simulink model "NonLin_BicycleModelSimulink"  (R2017b)
settings: Solver=VariableStepAuto  StartTime=0.0  StopTime=5  FixedStep=0.001  MaxStep=0.010  MinStep=0.005  RelTol=1e-3  EnableMultiTasking=on
values from neighbouring files (symbols this model uses):
  a = L*weight_dist    (= 0.762)    [BicycleModel.m]    (also in BicycleModelSim.m = 1.1; BicycleModelSimv2.m = 0.4572; FullCarModel.m = 0.6096; NonLin_BicycleModel.m = 0.8382)
  b = L*(1-weight_dist)    (= 0.762)    [BicycleModel.m]    (also in BicycleModelSim.m = 1.6; BicycleModelSimv2.m = 1.0668; FullCarModel.m = 0.9144; NonLin_BicycleModel.m = 0.6858)
  I_zz = 83.28    [BicycleModel.m]    (also in BicycleModelSim.m = 2500; BicycleModelSimv2.m; FullCarModel.m; NonLin_BicycleModel.m)
  m = 535*0.453592    (= 242.67172)    [BicycleModel.m]    (also in BicycleModelSim.m = 1500; BicycleModelSimv2.m = 242.6718; FullCarModel.m = 242.6718; NonLin_BicycleModel.m = 242.6718)
  step_steer = 1    [BicycleModelSimv2.m]    (also in FullCarModel.m = 0.0523598775598; NonLin_BicycleModel.m = 0.12217304764)
  weight_dist = 0.5    [BicycleModel.m]    (also in BicycleModelSimv2.m = 0.3; FullCarModel.m = 0.4; NonLin_BicycleModel.m = 0.55; ResponseTimePlotter.m = 0.51)
  X = cell2mat(Xbestcell)    [FullCarModel.m]    (also in NonLin_BicycleModel.m)
settings Model: Creator=tonylu  LastModifiedBy=tonylu
settings OptimizationCC: LifeSpan=inf
settings DebuggingCC: SFUnexpectedBacktrackingDiag=warning  SFNoUnconditionalDefaultTransitionDiag=warning  SFExecutionAtInitializationDiag=none
settings CodeAppCC: StateflowObjectComments=on
settings GRTTargetCC: TargetLangStandard=C89/C90 (ANSI)  GeneratePreprocessorConditionals=Disable all
settings ConfigComp: CovMetricSettings=dw  CovHtmlReporting=on  CovSaveCumulativeToWorkspaceVar=on  CovSaveSingleToWorkspaceVar=on  CovExternalEMLEnable=off

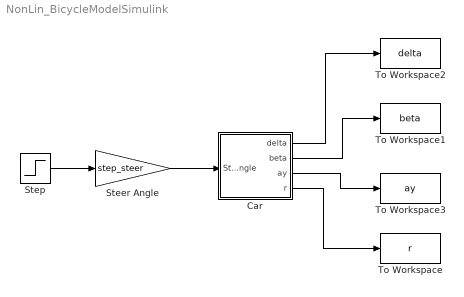
== system NonLin_BicycleModelSimulink ==
  Car : Subsystem
  Steer Angle : Gain  Gain=step_steer
  Step : Step  Time=0  SampleTime=0
  To Workspace : ToWorkspace  VariableName=r  SaveFormat=Structure With Time  SampleTime=0.01
  To Workspace1 : ToWorkspace  VariableName=beta  SaveFormat=Structure With Time  SampleTime=0.01
  To Workspace2 : ToWorkspace  VariableName=delta  SaveFormat=Structure With Time  SampleTime=0.01
  To Workspace3 : ToWorkspace  VariableName=ay  SaveFormat=Structure With Time  SampleTime=0.01
  wires:
  Car/1(delta) -> To Workspace2/1
  Car/2(beta) -> To Workspace1/1
  Car/3(ay) -> To Workspace3/1
  Car/4(r) -> To Workspace/1
  Steer Angle/1 -> Car/1(Steer Angle)
  Step/1 -> Steer Angle/1

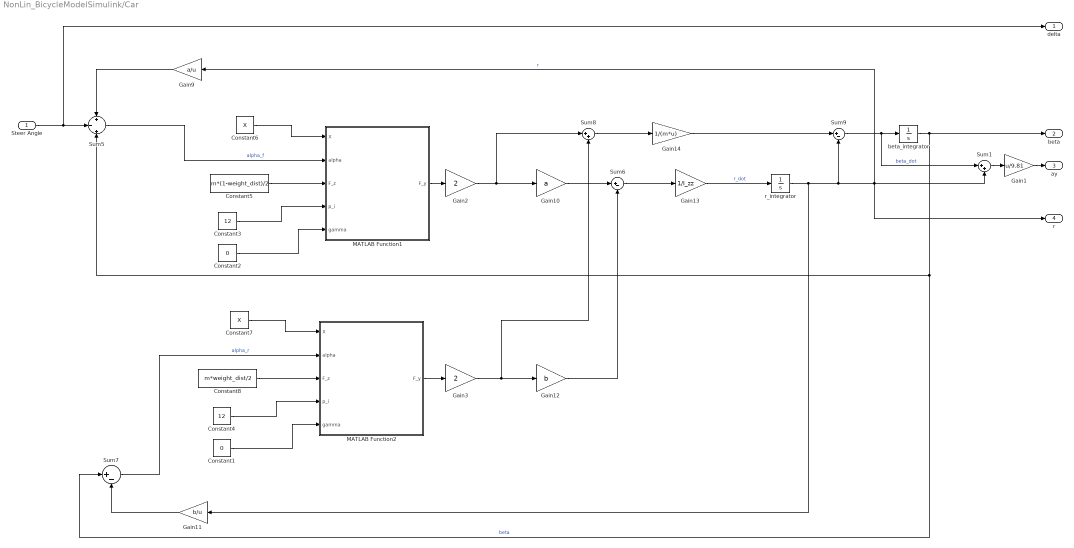
== system NonLin_BicycleModelSimulink/Car ==
  Steer Angle : Inport
  Constant1 : Constant  Value=0
  Constant2 : Constant  Value=0
  Constant3 : Constant  Value=12
  Constant4 : Constant  Value=12
  Constant5 : Constant  Value=m*(1-weight_dist)/2
  Constant6 : Constant  Value=X
  Constant7 : Constant  Value=X
  Constant8 : Constant  Value=m*weight_dist/2
  Gain1 : Gain  Gain=u/9.81
  Gain10 : Gain  Gain=a
  Gain11 : Gain  Gain=b/u
  Gain12 : Gain  Gain=b
  Gain13 : Gain  Gain=1/I_zz
  Gain14 : Gain  Gain=1/(m*u)
  Gain2 : Gain  Gain=2
  Gain3 : Gain  Gain=2
  Gain9 : Gain  Gain=a/u
  MATLAB Function1 : MATLAB Function  TreatAsAtomicUnit=on
  MATLAB Function2 : MATLAB Function  TreatAsAtomicUnit=on
  Sum1 : Sum  Inputs=|++
  Sum5 : Sum  Inputs=+|-|+
  Sum6 : Sum  Inputs=|+-
  Sum7 : Sum  Inputs=|+-
  Sum8 : Sum  Inputs=|++
  Sum9 : Sum  Inputs=|+-
  beta_integrator : Integrator
  r_integrator : Integrator
  delta : Outport
  beta : Outport  Port=2
  ay : Outport  Port=3
  r : Outport  Port=4
  wires:
  Steer Angle/1 -> delta/1, Sum5/2
  Gain9/1 -> Sum5/1
  Sum5/1 -> MATLAB Function1/2(alpha)  "alpha_f"
  Constant2/1 -> MATLAB Function1/5(gamma)
  Constant3/1 -> MATLAB Function1/4(p_i)
  Constant6/1 -> MATLAB Function1/1(X)
  r_integrator/1 -> Gain11/1, Sum9/2, Sum1/2, Gain9/1, r/1  "r"
  Gain10/1 -> Sum6/1
  Sum7/1 -> MATLAB Function2/2(alpha)  "alpha_r"
  Constant1/1 -> MATLAB Function2/5(gamma)
  Constant4/1 -> MATLAB Function2/4(p_i)
  Constant7/1 -> MATLAB Function2/1(X)
  MATLAB Function2/1(F_y) -> Gain3/1
  Gain11/1 -> Sum7/2
  beta_integrator/1 -> Sum7/1, Sum5/3, beta/1  "beta"
  Gain12/1 -> Sum6/2
  Sum6/1 -> Gain13/1
  Gain13/1 -> r_integrator/1  "r_dot"
  Sum8/1 -> Gain14/1
  Gain14/1 -> Sum9/1
  Sum9/1 -> Sum1/1, beta_integrator/1  "beta_dot"
  Sum1/1 -> Gain1/1
  Gain1/1 -> ay/1
  Constant8/1 -> MATLAB Function2/3(F_z)
  Constant5/1 -> MATLAB Function1/3(F_z)
  MATLAB Function1/1(F_y) -> Gain2/1
  Gain3/1 -> Sum8/2, Gain12/1
  Gain2/1 -> Sum8/1, Gain10/1

== matlab function NonLin_BicycleModelSimulink/Car/MATLAB Function1 ==
  data: X input; F_y output; alpha input; F_z input; p_i input; gamma input
function F_y  = lateralforce_pure(X,alpha,F_z,p_i,gamma)
%% Inputs
F_z = F_z/4.44822*9.81; % N to lbf

F_z0 = 200*ones(size(F_z)); %nominal load
p_i0 = 13*ones(size(p_i)); %nominal pressure

F_z = abs(F_z);

df_z = (F_z- F_z0)./F_z;
dp_i = (p_i-p_i0)./p_i;

%% Parameters

p_cy1 = X(1);
p_dy1 = X(2);
p_dy2 = X(3);
p_dy3 = X(4);
p_ey1 = X(5);
p_ey2 = X(6);
p_ey3 = X(7);
p_ey4 = X(8);
p_ey5 = X(9);
p_hy1 = X(10);
p_hy2 = X(11);
p_ky1 = X(12);
p_ky2 = X(13);
p_ky3 = X(14);
p_ky4 = X(15);
p_ky5 = X(16);
p_ky6 = X(17);
p_ky7 = X(18);
p_py1 = X(19);
p_py2 = X(20);
p_py3 = X(21);
p_py4 = X(22);
p_py5 = X(23);
p_vy1 = X(24);
p_vy2 = X(25);
p_vy3 = X(26);
p_vy4 = X(27);

%p_ey3 = 0
%p_dy1 = 1.8;
%p_dy2 = -0.05;

lambda_cy = 1;       % shape factor   
lambda_ey = 1;       % curvature 
lambda_hy = 0;       % horizontal shift
lambda_kyalpha = 1;  % cornering stiffness
lambda_kygamma = 1;  % camber force stiffness
lambda_muy = 0.55;      % peak friction coefficient
lambda_vy = 0;       % vertical shift

%%  Magic Formula Equations

K_yalpha = p_ky1.*F_z0.*(1+p_py1.*dp_i).*sin(p_ky4.*atan(F_z./...
    ((p_ky2 + p_ky5*gamma.^2).*(1+p_py2*dp_i).*F_z0))).*...
    (1-p_ky3.*abs(gamma)).*lambda_kyalpha;
K_ygamma = (p_ky6+p_ky7.*df_z).*(1+p_py5.*dp_i).*F_z.*lambda_kygamma;
S_vy0 = F_z.*(p_vy1+p_vy2.*df_z).*lambda_vy.*lambda_muy;
S_vygamma = F_z.*(p_vy3+p_vy4.*df_z).*gamma.*lambda_kygamma.*lambda_muy;
S_vy = S_vy0+S_vygamma;
S_hy0 = (p_hy1+p_hy2.*df_z).*lambda_hy;
S_hygamma = (K_ygamma.*gamma-S_vygamma)./K_yalpha;
S_hy = S_hy0+S_hygamma;
alpha_y = alpha+S_hy;
mu_y = (p_dy1+p_dy2.*df_z).*(1-p_dy3.*gamma.^2).*...
    (1+p_py3.*dp_i+p_py4.*dp_i.^2).*lambda_muy;
C_y = p_cy1.*lambda_cy;
D_y = mu_y.*F_z;
E_y = (p_ey1+p_ey2.*df_z).*(1+p_ey5.*gamma.^2-(p_ey3+p_ey4.*gamma).*sign(alpha_y)).*lambda_ey;
B_y = K_yalpha./C_y./D_y;

%Lateral Force
F_y = transpose(D_y.*sin(C_y.*atan(B_y.*alpha_y-E_y.*(B_y.*alpha_y-atan(B_y.*alpha_y))))+S_vy);

F_y = F_y*4.44822; % lbf to N

%F_y = -136*4.448*180/pi/2*alpha_y;

%F_y(F_z==0) = 0; %zero load

%F_y = K_yalpha*-0.0174533;

%F_y = -D_y

%F_y = mu_y;

end

== matlab function NonLin_BicycleModelSimulink/Car/MATLAB Function2 ==
  data: X input; F_y output; alpha input; F_z input; p_i input; gamma input
function F_y  = lateralforce_pure(X,alpha,F_z,p_i,gamma)
%% Inputs
F_z = F_z/4.44822*9.81; % N to lbf

F_z0 = 200*ones(size(F_z)); %nominal load
p_i0 = 13*ones(size(p_i)); %nominal pressure

F_z = abs(F_z);

df_z = (F_z- F_z0)./F_z;
dp_i = (p_i-p_i0)./p_i;

%% Parameters

p_cy1 = X(1);
p_dy1 = X(2);
p_dy2 = X(3);
p_dy3 = X(4);
p_ey1 = X(5);
p_ey2 = X(6);
p_ey3 = X(7);
p_ey4 = X(8);
p_ey5 = X(9);
p_hy1 = X(10);
p_hy2 = X(11);
p_ky1 = X(12);
p_ky2 = X(13);
p_ky3 = X(14);
p_ky4 = X(15);
p_ky5 = X(16);
p_ky6 = X(17);
p_ky7 = X(18);
p_py1 = X(19);
p_py2 = X(20);
p_py3 = X(21);
p_py4 = X(22);
p_py5 = X(23);
p_vy1 = X(24);
p_vy2 = X(25);
p_vy3 = X(26);
p_vy4 = X(27);

%p_ey3 = 0
%p_dy1 = 1.8;
%p_dy2 = -0.05;

lambda_cy = 1;       % shape factor   
lambda_ey = 1;       % curvature 
lambda_hy = 0;       % horizontal shift
lambda_kyalpha = 1;  % cornering stiffness
lambda_kygamma = 1;  % camber force stiffness
lambda_muy = 0.55;      % peak friction coefficient
lambda_vy = 0;       % vertical shift

%%  Magic Formula Equations

K_yalpha = p_ky1.*F_z0.*(1+p_py1.*dp_i).*sin(p_ky4.*atan(F_z./...
    ((p_ky2 + p_ky5*gamma.^2).*(1+p_py2*dp_i).*F_z0))).*...
    (1-p_ky3.*abs(gamma)).*lambda_kyalpha;
K_ygamma = (p_ky6+p_ky7.*df_z).*(1+p_py5.*dp_i).*F_z.*lambda_kygamma;
S_vy0 = F_z.*(p_vy1+p_vy2.*df_z).*lambda_vy.*lambda_muy;
S_vygamma = F_z.*(p_vy3+p_vy4.*df_z).*gamma.*lambda_kygamma.*lambda_muy;
S_vy = S_vy0+S_vygamma;
S_hy0 = (p_hy1+p_hy2.*df_z).*lambda_hy;
S_hygamma = (K_ygamma.*gamma-S_vygamma)./K_yalpha;
S_hy = S_hy0+S_hygamma;
alpha_y = alpha+S_hy;
mu_y = (p_dy1+p_dy2.*df_z).*(1-p_dy3.*gamma.^2).*...
    (1+p_py3.*dp_i+p_py4.*dp_i.^2).*lambda_muy;
C_y = p_cy1.*lambda_cy;
D_y = mu_y.*F_z;
E_y = (p_ey1+p_ey2.*df_z).*(1+p_ey5.*gamma.^2-(p_ey3+p_ey4.*gamma).*sign(alpha_y)).*lambda_ey;
B_y = K_yalpha./C_y./D_y;

%Lateral Force
F_y = transpose(D_y.*sin(C_y.*atan(B_y.*alpha_y-E_y.*(B_y.*alpha_y-atan(B_y.*alpha_y))))+S_vy);

F_y = F_y*4.44822; % lbf to N

%F_y = -136*4.448*180/pi/2*alpha_y;

%F_y(F_z==0) = 0; %zero load

%F_y = K_yalpha*-0.0174533;

%F_y = -D_y

%F_y = mu_y;

end
